simulink model "lyapunov_sim"  (R2021b)
settings: Solver=VariableStepAuto  StartTime=0.0  StopTime=10  RelTol=1e-3
settings Model: Creator=eraym  LastModifiedBy=eraym

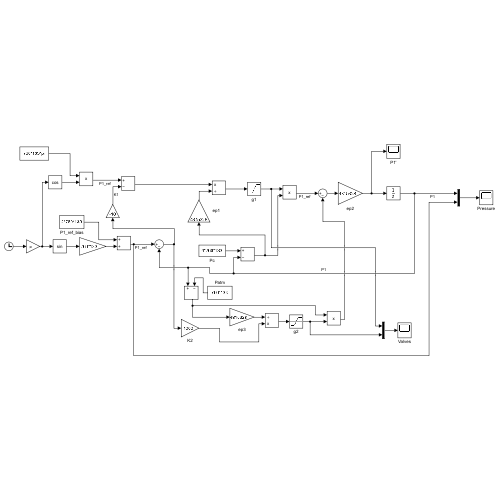
[thumbnail: Simulink's stored preview of the top-level diagram]
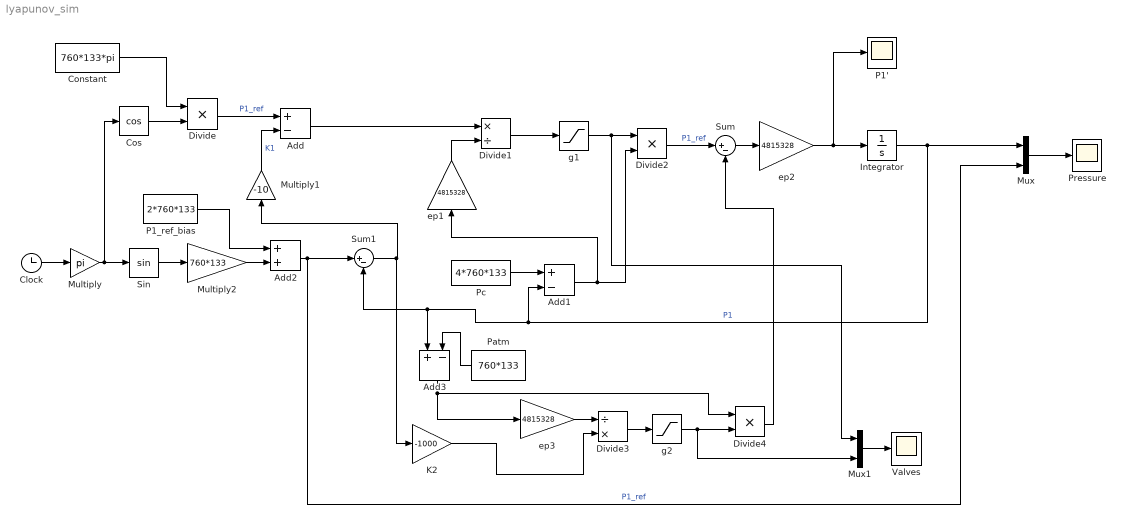
== system lyapunov_sim ==
  Add : Sum  Inputs=+-
  Add1 : Sum  Inputs=+-
  Add2 : Sum
  Add3 : Sum  Inputs=+-
  Clock : Clock
  Constant : Constant  Value=760*133*pi
  Cos : Trigonometry  Operator=cos
  Divide : Product  Inputs=**
  Divide1 : Product  Inputs=*/
  Divide2 : Product  Inputs=**
  Divide3 : Product  Inputs=/*
  Divide4 : Product  Inputs=**
  Integrator : Integrator  InitialCondition=1
  K2 : Gain  Gain=-1000
  Multiply : Gain  Gain=pi
  Multiply1 : Gain  Gain=-10
  Multiply2 : Gain  Gain=760*133
  Mux : Mux  Inputs=2
  Mux1 : Mux  Inputs=2
  P1' : Scope
  P1_ref_bias : Constant  Value=2*760*133
  Patm : Constant  Value=760*133
  Pc : Constant  Value=4*760*133
  Pressure : Scope
  Sin : Trigonometry
  Sum : Sum  Inputs=|+-
  Sum1 : Sum  Inputs=|+-
  Valves : Scope
  ep1 : Gain  Gain=4815328
  ep2 : Gain  Gain=4815328
  ep3 : Gain  Gain=4815328
  g1 : Saturate  UpperLimit=1  LowerLimit=-1
  g2 : Saturate  UpperLimit=1  LowerLimit=-1
  wires:
  Clock/1 -> Multiply/1
  Multiply/1 -> Sin/1, Cos/1
  Cos/1 -> Divide/2
  Constant/1 -> Divide/1
  Divide/1 -> Add/1  "P1_ref"
  Multiply1/1 -> Add/2  "K1"
  Add/1 -> Divide1/1
  ep1/1 -> Divide1/2
  Divide1/1 -> g1/1
  g1/1 -> Mux1/1, Divide2/1
  Divide2/1 -> Sum/1  "P1_ref"
  Sum/1 -> ep2/1
  ep2/1 -> P1'/1, Integrator/1
  Mux/1 -> Pressure/1
  Integrator/1 -> Sum1/2, Add3/1, Add1/2, Mux/1  "P1"
  Add1/1 -> ep1/1, Divide2/2
  Pc/1 -> Add1/1
  Sin/1 -> Multiply2/1
  Multiply2/1 -> Add2/2
  P1_ref_bias/1 -> Add2/1
  Add2/1 -> Sum1/1, Mux/2  "P1_ref"
  Sum1/1 -> K2/1, Multiply1/1
  K2/1 -> Divide3/2
  ep3/1 -> Divide3/1
  Add3/1 -> Divide4/1, ep3/1
  Patm/1 -> Add3/2
  Divide3/1 -> g2/1
  g2/1 -> Mux1/2, Divide4/2
  Divide4/1 -> Sum/2
  Mux1/1 -> Valves/1
